simulink model "FOC_Control_PMSM"  (R2024b)
settings: Solver=VariableStepAuto  StartTime=0.0  StopTime=2  RelTol=1e-3
undefined symbols (not defined in the file): pmsm, Ts
libraries: mcbcontrollergainlib x2, mcbfoclib x1, mcbpositiondecoderlib x1, slpidlib x1, mcbplantlib x1, autolibpmsminterior x1, mcbpmsmvflib x1
settings Model: Creator=ada09  LastModifiedBy=ada09

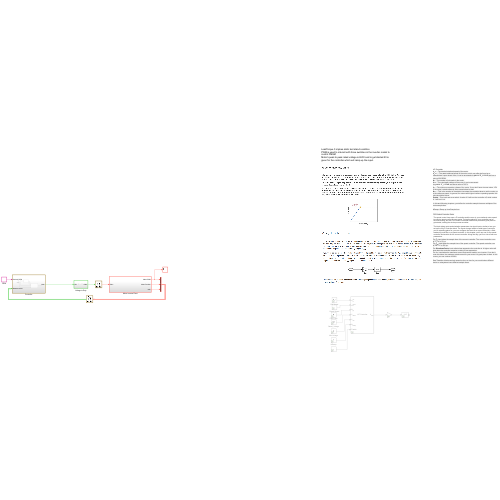
[thumbnail: Simulink's stored preview of the top-level diagram]
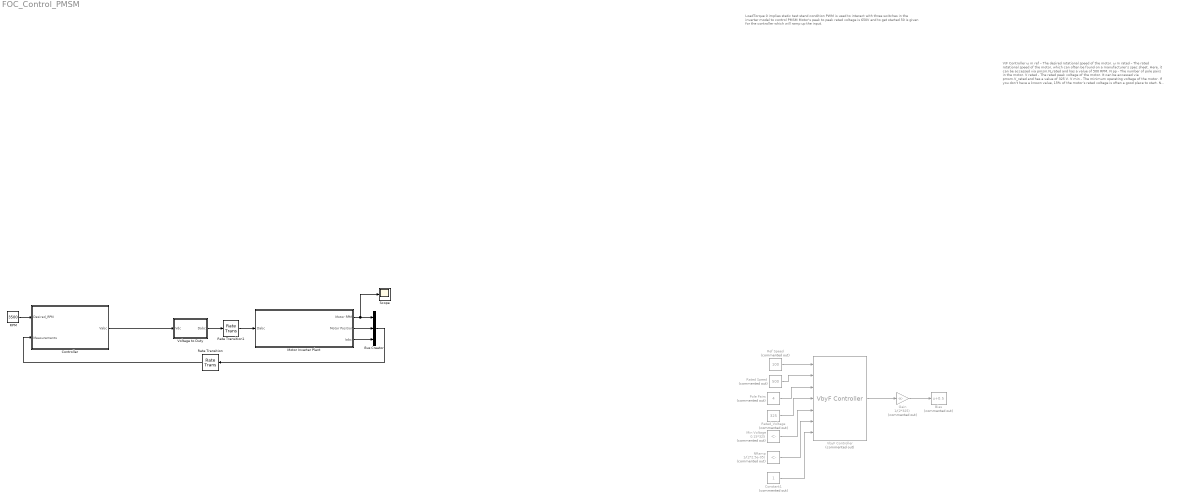
== system FOC_Control_PMSM ==
  note: V/F Controller
      | ω m ref – The desired rotational speed of the motor.
      | ω m rated – The rated rotational speed of the motor, which can often be found on a manufacturer’s spec sheet. Here, it can be accessed via pmsm.N_rated and has a value of 500 RPM.
      | N pp - The number of pole pairs in the motor.
      | V rated - The rated peak voltage of the motor. It can be accessed via pmsm.V_rated and has a value of 325 V.
      | V min - The minimum operating voltage of the motor. If you don’t have a known value, 15% of the motor’s rated voltage is often a good place to start.
      | N Ramp - This is the number of simulation time steps the controller takes to get the motor up to the reference speed. In general, for motors with higher inertia or operating speeds, this value should be higher.
      | Enable – This input acts as a switch. A value of 0 will turn the controller off, while a value of 1 will turn it on.
      |
      | In this and following chapters, you define the controller sample times as multiples of the motor sample time
      |
      | NRamp= Ramp up time/Sample time
      |
      | FOC Default Controller Gains
      | The speed control loop uses a PI controller and the error in your rotational motor speed to output a target current for your motor. Tuning the gains for your controller can be time-consuming, but the FOC Default Controller Gains block provides a good place to get started, making the whole process smoother.
      |
      | The block takes motor and simulation parameters via signal inputs, similar to how you set up the VbyF Controller block. The inputs change based on what type of controller you’re outputting gains for; you can configure the block for a current controller, a field-weakening controller, or a speed controller. In this chapter, you’ll use one for the speed controller and another for the current controller. Along the way, you’ll run into a few new parameters:
      |
      | The T S input takes the sample time of the current controller. The current controller runs at 2*Ts or 50 μs.
      | The T SC input takes the sample time of the speed controller. The speed controller runs at 20*Ts or 500 μs.
      | The SlowdownFactor input adjusts how aggressive the controller is. A higher value will slow down the controller response, making it less aggressive.
      | The I max input takes the maximum current that can be read by your inverter. If you don't know this value, the maximum rated current for your motor is a good place to start. In this course, you use a value of 200 A.
      |
      | Rate Transition blocks can help speed up the run time for your model when different blocks or subsystems have different sample times.
  note: LoadTorque 0 implies static test stand condition
      | PWM is used to interact with three switches in the inverter model to control PMSM
      | Motor's peak to peak rated voltage is 650V and to get started 50 is given for the controller which will ramp up the input.
  Bias : Bias  Commented=on  Bias=0.5  SaturateOnIntegerOverflow=off
  Bus Creator : BusCreator  Inputs=3
  Constant1 : Constant  Commented=on
  Controller : Subsystem
  Gain : Gain  Commented=on  Gain=1/(2*325)
  Min Voltage : Constant  Commented=on  Value=0.15*325
  Motor Inverter Plant : Subsystem
  NRamp : Constant  Commented=on  Value=1/(2*2.5e-05)
  Pole Pairs : Constant  Commented=on  Value=4
  RPM : Constant  Value=3500
  Rate Transition : RateTransition  OutPortSampleTime=2*Ts
  Rate Transition1 : RateTransition  OutPortSampleTime=Ts
  Rated Speed : Constant  Commented=on  Value=500
  Rated_Voltage : Constant  Commented=on  Value=325
  Ref Speed : Constant  Commented=on  Value=100
  Scope : Scope
  VbyF Controller : mcbpmsmvflib/VbyF Controller  Commented=on  SpeedUnit=RPM  BaseSpeed=1200  Ts=5e-05
      settings: LibrarySourceBlock=mcblib/Controls/Controllers/VbyF Controller
  Voltage to Duty : Subsystem
  wires:
  Ref Speed/1 -> VbyF Controller/1
  Rated Speed/1 -> VbyF Controller/2
  Pole Pairs/1 -> VbyF Controller/3
  Rated_Voltage/1 -> VbyF Controller/4
  Min Voltage/1 -> VbyF Controller/5
  NRamp/1 -> VbyF Controller/6
  Constant1/1 -> VbyF Controller/7
  VbyF Controller/1 -> Gain/1
  Gain/1 -> Bias/1
  Motor Inverter Plant/1(Motor RPM) -> Scope/1, Bus Creator/1
  Motor Inverter Plant/2(Motor Position) -> Bus Creator/2
  Motor Inverter Plant/3(Iabc) -> Bus Creator/3
  Voltage to Duty/1(Dabc) -> Rate Transition1/1
  Bus Creator/1 -> Rate Transition/1
  Controller/1(Vabc) -> Voltage to Duty/1(Vdc)
  RPM/1 -> Controller/1(Desired_RPM)
  Rate Transition/1 -> Controller/2(Measurements)
  Rate Transition1/1 -> Motor Inverter Plant/1(Dabc)

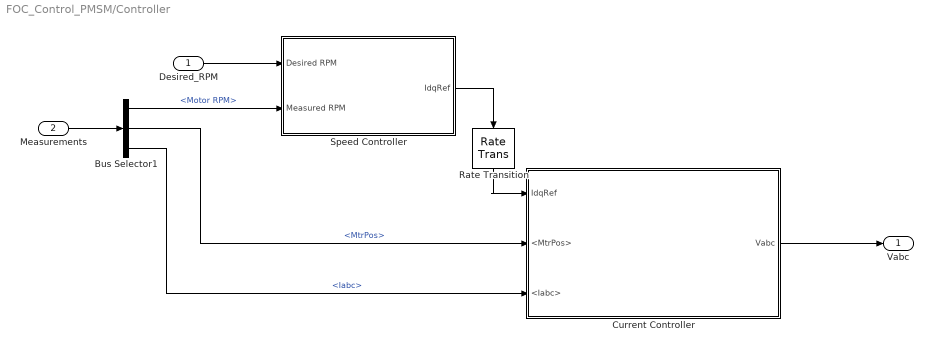
== system FOC_Control_PMSM/Controller ==
  Desired_RPM : Inport
  Measurements : Inport  Port=2
  Bus Selector1 : BusSelector  OutputSignals=Motor RPM,MtrPos,Iabc
  Current Controller : Subsystem
  Rate Transition : RateTransition  OutPortSampleTime=2*Ts
  Speed Controller : Subsystem
  Vabc : Outport
  wires:
  Measurements/1 -> Bus Selector1/1
  Bus Selector1/1 -> Speed Controller/2(Measured RPM)  "<Motor RPM>"
  Speed Controller/1(IdqRef) -> Rate Transition/1
  Desired_RPM/1 -> Speed Controller/1(Desired RPM)
  Bus Selector1/3 -> Current Controller/3(<Iabc>)  "<Iabc>"
  Bus Selector1/2 -> Current Controller/2(<MtrPos>)  "<MtrPos>"
  Current Controller/1(Vabc) -> Vabc/1
  Rate Transition/1 -> Current Controller/1(IdqRef)

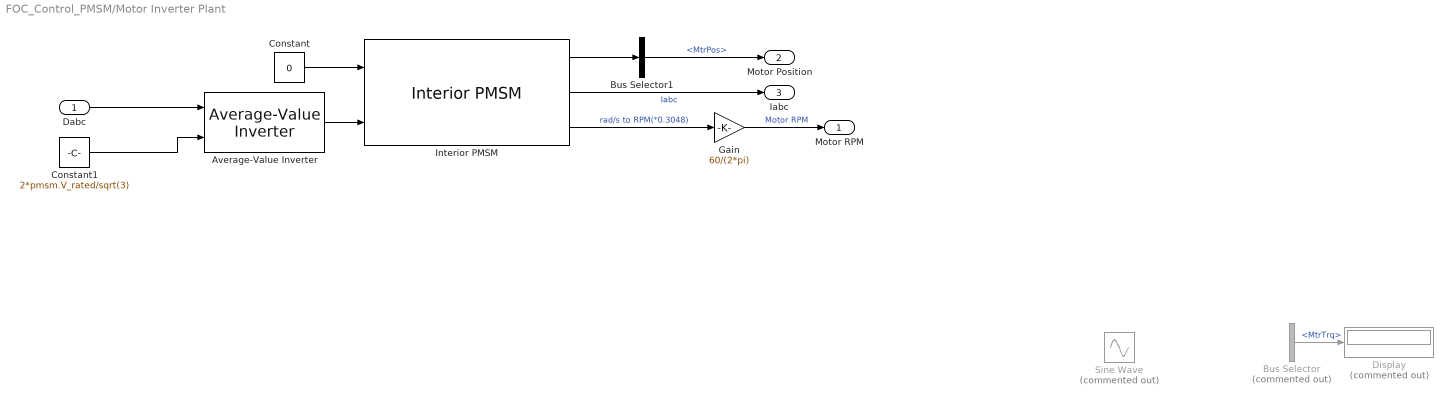
== system FOC_Control_PMSM/Motor Inverter Plant ==
  Dabc : Inport
  Average-Value Inverter : mcbplantlib/Average-Value Inverter
      settings: LibrarySourceBlock=mcblib/Electrical Systems/Inverters/Average-Value Inverter
  Bus Selector : BusSelector  Commented=on  OutputSignals=MtrTrq
  Bus Selector1 : BusSelector  OutputSignals=MtrPos
  Constant : Constant  Value=0
  Constant1 : Constant  Value=2*pmsm.V_rated/sqrt(3)
  Display : Display  Commented=on
  Gain : Gain  Gain=60/(2*pi)
  Interior PMSM : autolibpmsminterior/Interior PMSM  port_config=Torque  sim_type=Discrete  Ts=Ts  P=pmsm.p  Rs=pmsm.Rs  Ldq=[pmsm.Ld, pmsm.Lq]  KConstText=Permanent flux linkage constant (lambda_pm):  lambda_pm=pmsm.FluxPM  Ke=159.9771  mechanical=[pmsm.J, 0, 0]  idq0=[0 0]  theta_init=0  omega_init=0  KConst=pmsm.FluxPM  lambda_pm_calc=pmsm.FluxPM  Kt=0.07  RefBlkName='autolibpmsminterior/Interior PMSM'  aMode=5
      settings: LibrarySourceBlock=mcblib/Electrical Systems/Motors/Interior PMSM
  Sine Wave : Sin  Commented=on  Bias=0.5  Frequency=120  Phase=[0 -2*pi/3 -4*pi/3]  SampleTime=0
  Motor RPM : Outport
  Motor Position : Outport  Port=2
  Iabc : Outport  Port=3
  wires:
  Interior PMSM/2 -> Iabc/1  "Iabc"
  Constant1/1 -> Average-Value Inverter/2
  Average-Value Inverter/1 -> Interior PMSM/2
  Bus Selector/1 -> Display/1  "<MtrTrq>"
  Interior PMSM/3 -> Gain/1  "rad/s to RPM(*0.3048)"
  Constant/1 -> Interior PMSM/1
  Gain/1 -> Motor RPM/1  "Motor RPM"
  Dabc/1 -> Average-Value Inverter/1
  Interior PMSM/1 -> Bus Selector1/1
  Bus Selector1/1 -> Motor Position/1  "<MtrPos>"

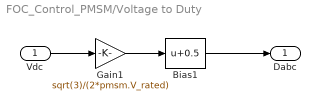
== system FOC_Control_PMSM/Voltage to Duty ==
  Vdc : Inport
  Bias1 : Bias  Bias=0.5  SaturateOnIntegerOverflow=off
  Gain1 : Gain  Gain=sqrt(3)/(2*pmsm.V_rated)
  Dabc : Outport
  wires:
  Gain1/1 -> Bias1/1
  Vdc/1 -> Gain1/1
  Bias1/1 -> Dabc/1

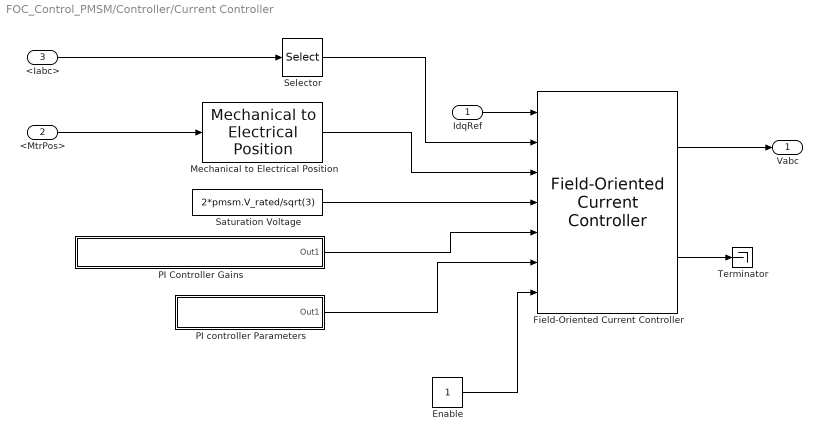
== system FOC_Control_PMSM/Controller/Current Controller ==
  IdqRef : Inport
  <MtrPos> : Inport  Port=2
  <Iabc> : Inport  Port=3
  Enable : Constant
  Field-Oriented Current Controller : mcbfoclib/Field-Oriented Current Controller  AngleUnit=Radians  NumberOfLUTPoints=1024  AxisAlignment=D-axis  SaturationMethod=D-Q equivalence  PWMMethod=SVM: space vector modulation
      settings: LibrarySourceBlock=mcblib/Controls/Controllers/Field-Oriented Current Controller
  Mechanical to Electrical Position : mcbpositiondecoderlib/Mechanical to Electrical Position  PolePairsInputType=Specify via dialog  NrPP=pmsm.p  selectedRange=Radians  MechOfstInputType=Specify via dialog  mechOffsetIn=0  maxAngleIn=2*pi  InputDataType=single  VariantSelect=floating-point
      settings: LibrarySourceBlock=mcblib/Sensor Decoders/Mechanical to Electrical Position
  PI Controller Gains : Subsystem
  PI controller Parameters : Subsystem
  Saturation Voltage : Constant  Value=2*pmsm.V_rated/sqrt(3)
  Selector : Selector  InputPortWidth=3  IndexOptions=Index vector (dialog)  Indices=[1 2]  OutputSizes=1
  Terminator : Terminator
  Vabc : Outport
  wires:
  Mechanical to Electrical Position/1 -> Field-Oriented Current Controller/3
  Enable/1 -> Field-Oriented Current Controller/7
  <Iabc>/1 -> Selector/1
  Saturation Voltage/1 -> Field-Oriented Current Controller/4
  PI controller Parameters/1(Out1) -> Field-Oriented Current Controller/6
  PI Controller Gains/1(Out1) -> Field-Oriented Current Controller/5
  Selector/1 -> Field-Oriented Current Controller/2
  <MtrPos>/1 -> Mechanical to Electrical Position/1
  Field-Oriented Current Controller/1 -> Vabc/1
  IdqRef/1 -> Field-Oriented Current Controller/1
  Field-Oriented Current Controller/2 -> Terminator/1

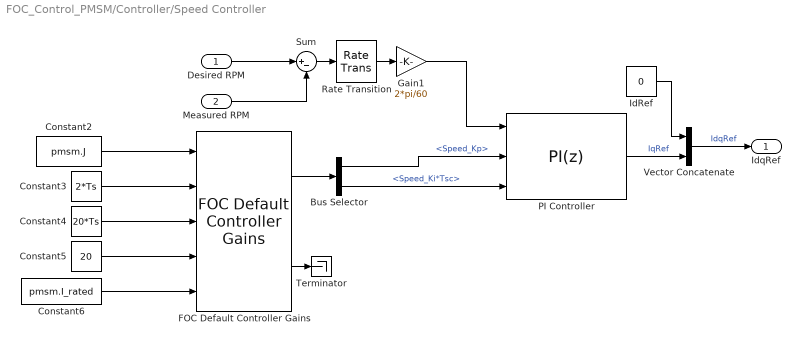
== system FOC_Control_PMSM/Controller/Speed Controller ==
  Desired RPM : Inport
  Measured RPM : Inport  Port=2
  Bus Selector : BusSelector  OutputSignals=Speed_Kp,Speed_Ki*Tsc
  Constant2 : Constant  Value=pmsm.J
  Constant3 : Constant  Value=2*Ts
  Constant4 : Constant  Value=20*Ts
  Constant5 : Constant  Value=20
  Constant6 : Constant  Value=pmsm.I_rated
  FOC Default Controller Gains : mcbcontrollergainlib/FOC Default Controller Gains  motorSelection=PMSM  unitType=SI Unit  outCurrentControlGain=off  outFWCGain=off  outSpeedControlGain=on  externalDelay=off  currentSensorDelay=50e-6  speedSensorDelay=50e-6  speedFilterDelay=0.02
      settings: LibrarySourceBlock=mcblib/Controls/Controllers/FOC Default Controller Gains
  Gain1 : Gain  Gain=2*pi/60
  IdRef : Constant  Value=0
  PI Controller : slpidlib/PID Controller  Controller=PI  Form=Parallel  TimeDomain=Discrete-time  UseExternalTs=off  SampleTime=-1  IntegratorMethod=Forward Euler  FilterMethod=Forward Euler  ControllerParametersSource=external  P=1  I=1  UseKiTs=on  D=0  UseExternalDerivativeSource=off  N=100  UseFilter=on  TunerSelectOption=Transfer Function Based (PID Tuner App)  InitialConditionSource=internal  InitialConditionForIntegrator=0  InitialConditionForFilter=0  DifferentiatorICPrevScaledInput=0  ExternalReset=none  TrackingMode=off  Kt=1  LimitOutput=on  SatLimitsSource=internal  UpperSaturationLimit=pmsm.I_rated  LowerSaturationLimit=-pmsm.I_rated  LinearizeAsGain=on  AntiWindupMode=clamping  Kb=1  LimitIntegrator=on  UpperIntegratorSaturationLimit=pmsm.I_rated  LowerIntegratorSaturationLimit=-pmsm.I_rated  RndMeth=Simplest  POutMin=[]  POutMax=[]  IOutMin=[]  IOutMax=[]  DOutMin=[]  DOutMax=[]  NOutMin=[]  NOutMax=[]  SumOutMin=[]  SumOutMax=[]  SaturationOutDataTypeStr=Inherit: Inherit via back propagation  SaturationOutMin=[]  SaturationOutMax=[]  PParamMin=[]  PParamMax=[]  IParamMin=[]  IParamMax=[]  DParamMin=[]  DParamMax=[]  NParamMin=[]  NParamMax=[]  KbParamMin=[]  KbParamMax=[]  KtParamMin=[]  KtParamMax=[]  KbOutMin=[]  KbOutMax=[]  KtOutMin=[]  KtOutMax=[]  IntegratorOutMin=[]  IntegratorOutMax=[]  FilterOutMin=[]  FilterOutMax=[]  SumI1OutMin=[]  SumI1OutMax=[]  SumI2OutMin=[]  SumI2OutMax=[]  SumI3OutMin=[]  SumI3OutMax=[]  SumI4OutMin=[]  SumI4OutMax=[]  SumDOutMin=[]  SumDOutMax=[]  DifferentiatorOutMin=[]  DifferentiatorOutMax=[]  FilterDiffOutCoefMin=[]  FilterDiffOutCoefMax=[]  ReciprocalOutMin=[]  ReciprocalOutMax=[]  SumDenOutMin=[]  SumDenOutMax=[]  SumNumOutMin=[]  SumNumOutMax=[]  DivideOutMin=[]  DivideOutMax=[]  UdiffTsProdOutMin=[]  UdiffTsProdOutMax=[]  NTsProdOutMin=[]  NTsProdOutMax=[]  UintegralTsProdOutMin=[]  UintegralTsProdOutMax=[]  UngainTsProdOutMin=[]  UngainTsProdOutMax=[]  ClampingZeroOutDataTypeStr=Inherit: Inherit via back propagation  ClampingZeroOutMin=[]  ClampingZeroOutMax=[]  FilterDenConstantOutDataTypeStr=Inherit: Inherit via back propagation  FilterDenConstantOutMin=[]  FilterDenConstantOutMax=[]  PCopyOutDataTypeStr=Inherit: Inherit via back propagation  PCopyOutMin=[]  PCopyOutMax=[]  NCopyOutDataTypeStr=Inherit: Inherit via back propagation  NCopyOutMin=[]  NCopyOutMax=[]  IntegratorContinuousStateAttributes=''  IntegratorStateMustResolveToSignalObject=off  IntegratorRTWStateStorageClass=Auto  FilterContinuousStateAttributes=''  FilterStateMustResolveToSignalObject=off  FilterRTWStateStorageClass=Auto  ParallelPVariant=ExternalParameters  IdealPVariant=Disabled  IVariant=ExternalParameters  DVariant=Disabled  IntegratorVariant=Discrete  SatVariant=Enabled  AWVariant=DiscClampingParallel  PCopyVariant=Disabled  TRVariant=Disabled  FdbkBlocksVariant=Forward  IdealPFdbkVariant=Disabled  SatFdbkVariant=Disabled  DerivativeFilterVariant=Disabled  NVariant=Disabled  NCopyVariant=Disabled_SignalSpec  FilterICVariant=Disabled  IntegratorICVariant=InternalICs  ExternalResetVariant=Disabled  TRSumVariant=Passthrough  SumFdbkVariant=Disabled  SumVariant=Sum_PI  TsampFilterVariant=InternalTs  TsampNgainVariant=Passthrough  TsampIntegralVariant=Disabled_SignalSpec  ExternalSaturationOutDataTypeStr=Inherit: Same as second input  DerivativeSourceVariant=Disabled  PreIntVariant=InternalPreInt
      settings: LibrarySourceBlock=mcblib/Controls/Controllers/PI Controller
  Rate Transition : RateTransition  OutPortSampleTime=20*Ts
  Sum : Sum  Inputs=|+-
  Terminator : Terminator
  Vector Concatenate : Concatenate
  IdqRef : Outport
  wires:
  Constant5/1 -> FOC Default Controller Gains/4
  FOC Default Controller Gains/2 -> Terminator/1
  Measured RPM/1 -> Sum/2
  Constant2/1 -> FOC Default Controller Gains/1
  PI Controller/1 -> Vector Concatenate/2  "IqRef"
  Vector Concatenate/1 -> IdqRef/1  "IdqRef"
  Bus Selector/1 -> PI Controller/2  "<Speed_Kp>"
  Constant6/1 -> FOC Default Controller Gains/5
  Gain1/1 -> PI Controller/1
  FOC Default Controller Gains/1 -> Bus Selector/1
  Constant3/1 -> FOC Default Controller Gains/2
  Constant4/1 -> FOC Default Controller Gains/3
  Bus Selector/2 -> PI Controller/3  "<Speed_Ki*Tsc>"
  IdRef/1 -> Vector Concatenate/1
  Desired RPM/1 -> Sum/1
  Sum/1 -> Rate Transition/1
  Rate Transition/1 -> Gain1/1

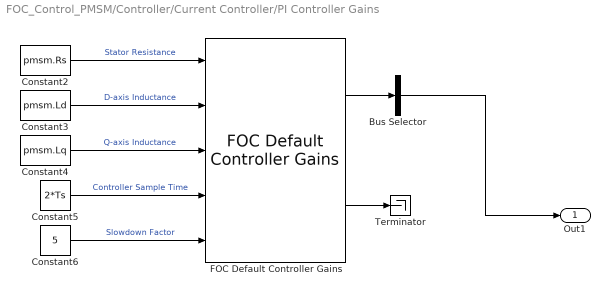
== system FOC_Control_PMSM/Controller/Current Controller/PI Controller Gains ==
  Bus Selector : BusSelector  OutputSignals=Daxis_Kp,Daxis_Ki*Ts,Qaxis_Kp,Qaxis_Ki*Ts  OutputAsBus=on
  Constant2 : Constant  Value=pmsm.Rs
  Constant3 : Constant  Value=pmsm.Ld
  Constant4 : Constant  Value=pmsm.Lq
  Constant5 : Constant  Value=2*Ts
  Constant6 : Constant  Value=5
  FOC Default Controller Gains : mcbcontrollergainlib/FOC Default Controller Gains  motorSelection=PMSM  unitType=SI Unit  outCurrentControlGain=on  outFWCGain=off  outSpeedControlGain=off  externalDelay=off  currentSensorDelay=50e-6  speedSensorDelay=50e-6  speedFilterDelay=0.02
      settings: LibrarySourceBlock=mcblib/Controls/Controllers/FOC Default Controller Gains
  Terminator : Terminator
  Out1 : Outport
  wires:
  Bus Selector/1 -> Out1/1
  Constant4/1 -> FOC Default Controller Gains/3  "Q-axis Inductance"
  FOC Default Controller Gains/2 -> Terminator/1
  FOC Default Controller Gains/1 -> Bus Selector/1
  Constant6/1 -> FOC Default Controller Gains/5  "Slowdown Factor"
  Constant3/1 -> FOC Default Controller Gains/2  "D-axis Inductance"
  Constant5/1 -> FOC Default Controller Gains/4  "Controller Sample Time"
  Constant2/1 -> FOC Default Controller Gains/1  "Stator Resistance"

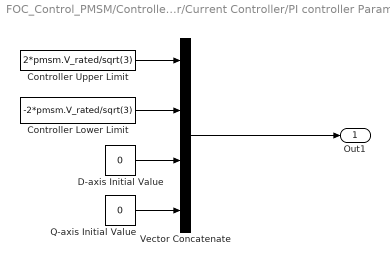
== system FOC_Control_PMSM/Controller/Current Controller/PI controller Parameters ==
  Controller Lower Limit : Constant  Value=-2*pmsm.V_rated/sqrt(3)
  Controller Upper Limit : Constant  Value=2*pmsm.V_rated/sqrt(3)
  D-axis Initial Value : Constant  Value=0
  Q-axis Initial Value : Constant  Value=0
  Vector Concatenate : Concatenate  NumInputs=4
  Out1 : Outport
  wires:
  Q-axis Initial Value/1 -> Vector Concatenate/4
  Controller Upper Limit/1 -> Vector Concatenate/1
  Vector Concatenate/1 -> Out1/1
  Controller Lower Limit/1 -> Vector Concatenate/2
  D-axis Initial Value/1 -> Vector Concatenate/3
